simulink model "mech_four_bar_lin"  (Simulink 6.0)
settings: Solver=ode45  StartTime=0.0  StopTime=10.0  RelTol=1e-3  AbsTol=1e-6
PreLoadFcn:
  | alpha = 60*pi/180; beta = 149.5*pi/180;
  | gamma = 54.8*pi/180; delta = 95.7*pi/180;
  | beta2 = beta + alpha - pi; delta2 = pi - delta;
  | len1 = 0.59; len2 = 1; len3 = 0.11; len4 = 0.867;
libraries: mblibv1 x11
Description:
  | Linearization example: four-bar mechanism, closed-loop topology.
settings Model: Creator=arnav  LastModifiedBy=batserve  ExtModeAutoUpdateStatusClock=off
settings SolverCC: MaxOrder=1
settings DataIOCC: SaveState=on  SignalLoggingName=sigsOut  Refine=5
settings OptimizationCC: BooleanDataType=off
settings DebuggingCC: CheckExecutionContextPreStartOutputMsg=on  CheckExecutionContextRuntimeOutputMsg=on  SolverPrmCheckMsg=none  UnconnectedInputMsg=none  UnconnectedOutputMsg=none  UnconnectedLineMsg=none
settings HardwareCC: TargetUnknown=on
settings ModelReferenceCC: UpdateModelReferenceTargets=IfOutOfDate
settings SimMechanicsCC: VisOnUpdateDiagram=on  VisDuringSimulation=on

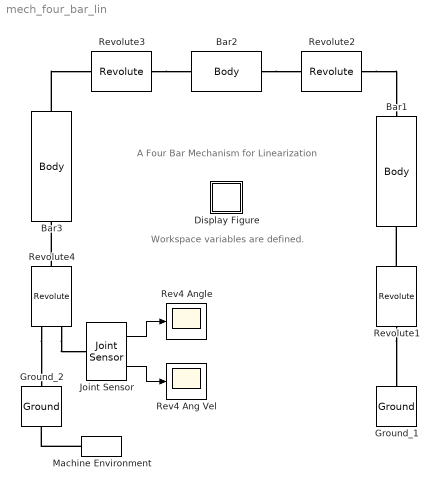
== system mech_four_bar_lin ==
  note: A Four Bar Mechanism
      | for Linearization
  note: Workspace variables
      | are defined.
  Bar1 : mblibv1/Bodies/Body  Orientation=down  PhysicalDomain=mechanical  SubClassName=Unknown  LeftPortType=workingframe  RightPortType=workingframe  LConnTagsString=CS1  RConnTagsString=CS2  DialogClass=MechanicalBodyBlock  Mass=5.357  MassUnits=kg  InertiaUnits=kg*m^2  Inertia=[1.07e-3 0 0;0 0.143 0;0 0 0.143]  Shape=Cylinder  ShapeDims=[1 1]  ShapeUnits=m  ShapeUse=false  Density=1  DensityUnits=kg/m^3  DensityUse=false  CG=Left$CG$(len1/2)*[cos(delta2) sin(delta2) 0]$WORLD$CS2$m$[0 0 delta2]$Euler X-Y-Z$rad$WORLD$false  WorkingFrames=Left$CS1$len1*[cos(delta2) sin(delta2) 0]$WORLD$CS2$m$[0 0 0]$Euler X-Y-Z$deg$WORLD$true#Right$CS2$[0 0 0]$WORLD$ADJOINING$m$[0 0 0]$Euler X-Y-Z$deg$WORLD$true
  Bar2 : mblibv1/Bodies/Body  PhysicalDomain=mechanical  SubClassName=Unknown  LeftPortType=workingframe  RightPortType=workingframe  LConnTagsString=CS1  RConnTagsString=CS2  DialogClass=MechanicalBodyBlock  Mass=9.028  MassUnits=kg  InertiaUnits=kg*m^2  Inertia=[1.8e-3 0 0;0 0.678 0;0 0 0.678]  Shape=Cylinder  ShapeDims=[1 1]  ShapeUnits=m  ShapeUse=false  Density=1  DensityUnits=kg/m^3  DensityUse=false  CG=Left$CG$(len2/2)*[cos(beta2) sin(beta2) 0]$WORLD$CS1$m$[0 0 beta2]$Euler X-Y-Z$rad$WORLD$false  WorkingFrames=Left$CS1$[0 0 0]$WORLD$ADJOINING$m$[0 0 0]$Euler X-Y-Z$deg$WORLD$true#Right$CS2$(len2)*[cos(beta2) sin(beta2) 0]$WORLD$CS1$m$[0 0 0]$Euler X-Y-Z$deg$WORLD$true
  Bar3 : mblibv1/Bodies/Body  Orientation=up  PhysicalDomain=mechanical  SubClassName=Unknown  LeftPortType=workingframe  RightPortType=workingframe  LConnTagsString=CS1  RConnTagsString=CS2  DialogClass=MechanicalBodyBlock  Mass=0.991  MassUnits=kg  InertiaUnits=kg*m^2  Inertia=[2.06e-4 0 0;0 1.1e-3 0;0 0 1.1e-3]  Shape=Cylinder  ShapeDims=[1 1]  ShapeUnits=m  ShapeUse=false  Density=1  DensityUnits=kg/m^3  DensityUse=false  CG=Left$CG$(len3/2)*[cos(alpha) sin(alpha) 0]$WORLD$CS1$m$[0 0 alpha]$Euler X-Y-Z$rad$WORLD$false  WorkingFrames=Left$CS1$[0 0 0]$WORLD$ADJOINING$m$[0 0 0]$Euler X-Y-Z$deg$WORLD$true#Right$CS2$len3*[cos(alpha) sin(alpha) 0]$WORLD$CS1$m$[0 0 0]$Euler X-Y-Z$deg$WORLD$true
  Display Figure : Subsystem  Tag=Help  Description="Help callback for linearized four bar model: mech_four_bar_lin.  Opens Help browser to Type 19 marker at documentation for this tutorial model."
      settings: OpenFcn=pmhelpview([docroot '/toolbox/physmod/mech/mech.map'], 'mech_four_bar_lin_help');
      mask Type: Help callback
      mask Display: image(imread('info.bmp'))
  Ground_1 : mblibv1/Bodies/Ground  Orientation=up  Opaque=on  LeftPortType=env  RightPortType=workingframe  PhysicalDomain=Mechanical  DialogClass=GroundBlock  CoordPosition=[0.433 0.04 0]  CoordPositionUnits=m  StateVectorMgrId=-1  MachineId=[0 0]  ShowEnvPort=off
  Ground_2 : mblibv1/Bodies/Ground  Orientation=up  Opaque=on  LeftPortType=env  RightPortType=workingframe  PhysicalDomain=Mechanical  DialogClass=GroundBlock  CoordPosition=[-0.434 0.04 0]  CoordPositionUnits=m  StateVectorMgrId=-1  MachineId=[0 0]  ShowEnvPort=on
  Joint Sensor : mblibv1/Sensors &  Actuators/Joint Sensor  Opaque=on  PhysicalDomain=Mechanical  PortType=blob  Muxed=off  Pose=on  Angle=on  AngleUnits=deg  ArcVelocity=on  ArcVelocityUnits=deg/s  ArcAcceleration=off  ArcAccelerationUnits=deg/s^2  CoordPosition=on  CoordPositionUnits=m  Velocity=off  VelocityUnits=m/s  Acceleration=off  AccelerationUnits=m/s^2  Quaternion=on  QuaternionDT=off  QuaternionDDT=off  QuaternionUnits=off  OutputVector=[ 1 1 ]  ActiveIO=on  Width=2  DialogClass=MechanicalSensorBlock  Primitive=R1  Force=off  ForceUnits=N  Torque=off  TorqueUnits=N-m  ReferenceFrame=Absolute (INERTIAL)  ReactionSensedSide=Base  ReactionReferenceFrame=Absolute (World)  ReactionForce=off  ReactionForceUnits=N  ReactionMoment=off  ReactionMomentUnits=N-m
  Machine Environment : mblibv1/Bodies/Machine Environment  Tag=Factory ground  Orientation=left  DialogController=MECH.DialogSource  Opaque=on  PortType=env  PhysicalDomain=Mechanical  DialogTemplateClass=MECH.MachineEnvironment  SyncWhenCopied=off  Gravity=[0 -9.81 0]  GravityUnits=m/s^2  GravityAsSignal=off  Dimensionality=3D Only  AnalysisType=Forward dynamics  LinearAssemblyTolerance=1e-3  LinearAssemblyToleranceUnits=m  AngularAssemblyTolerance=1e-3  AngularAssemblyToleranceUnits=rad  ConstraintSolverType=Stabilizing  ConstraintRelTolerance=1e-4  ConstraintAbsTolerance=1e-4  UseRobustSingularityHandling=off  StatePerturbationType=Adaptive  PerturbationSize=1e-3  VisualizeMachine=on
  Rev4 Ang Vel : Scope
      settings: TimeRange=10  YMin=-125  YMax=125  SaveName=ScopeData2
  Rev4 Angle : Scope
      settings: TimeRange=10  YMin=-27.5  YMax=2.5
  Revolute1 : mblibv1/Joints/Revolute  Orientation=down  PhysicalDomain=mechanical  SubClassName=Unknown  LeftPortType=blob  RightPortType=blob  LConnTagsString=__newl0  RConnTagsString=__newr0  NumSAPorts=0  CutJoint=on  MarkAsCut=off  Primitives=revolute  PrimitiveProps=R1$WORLD$[0 0 1]$revolute  DialogClass=JointBlock
  Revolute2 : mblibv1/Joints/Revolute  PhysicalDomain=mechanical  SubClassName=Unknown  LeftPortType=blob  RightPortType=blob  LConnTagsString=__newl0  RConnTagsString=__newr0  NumSAPorts=0  CutJoint=off  MarkAsCut=off  Primitives=revolute  PrimitiveProps=R1$WORLD$[0 0 1]$revolute  DialogClass=JointBlock
  Revolute3 : mblibv1/Joints/Revolute  PhysicalDomain=mechanical  SubClassName=Unknown  LeftPortType=blob  RightPortType=blob  LConnTagsString=__newl0  RConnTagsString=__newr0  NumSAPorts=0  CutJoint=off  MarkAsCut=off  Primitives=revolute  PrimitiveProps=R1$WORLD$[0 0 1]$revolute  DialogClass=JointBlock
  Revolute4 : mblibv1/Joints/Revolute  Orientation=up  PhysicalDomain=mechanical  SubClassName=Unknown  LeftPortType=blob  RightPortType=blob  LConnTagsString=__newl0|SA1  RConnTagsString=__newr0  NumSAPorts=1  CutJoint=off  MarkAsCut=off  Primitives=revolute  PrimitiveProps=R1$WORLD$[0 0 1]$revolute  DialogClass=JointBlock
  wires:
  Joint Sensor/1 -> Rev4 Angle/1
  Joint Sensor/2 -> Rev4 Ang Vel/1
  connections:
  Revolute4/RConn1 -- Bar3/LConn1
  Revolute4/LConn1 -- Ground_2/RConn1
  Revolute4/LConn2 -- Joint Sensor/LConn1
  Bar3/RConn1 -- Revolute3/LConn1
  Revolute3/RConn1 -- Bar2/LConn1
  Bar2/RConn1 -- Revolute2/LConn1
  Revolute2/RConn1 -- Bar1/LConn1
  Revolute1/LConn1 -- Bar1/RConn1
  Revolute1/RConn1 -- Ground_1/RConn1
  Machine Environment/RConn1 -- Ground_2/LConn1

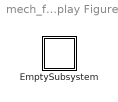
== system mech_four_bar_lin/Display Figure ==
  EmptySubsystem : Subsystem

== system mech_four_bar_lin/Display Figure/EmptySubsystem ==
